simulink model "Modelka_3"  (Simulink 4.00)
settings: Solver=ode45  StartTime=0.0  StopTime=10.0  RelTol=1e-3
settings Model: LastModifiedBy=user

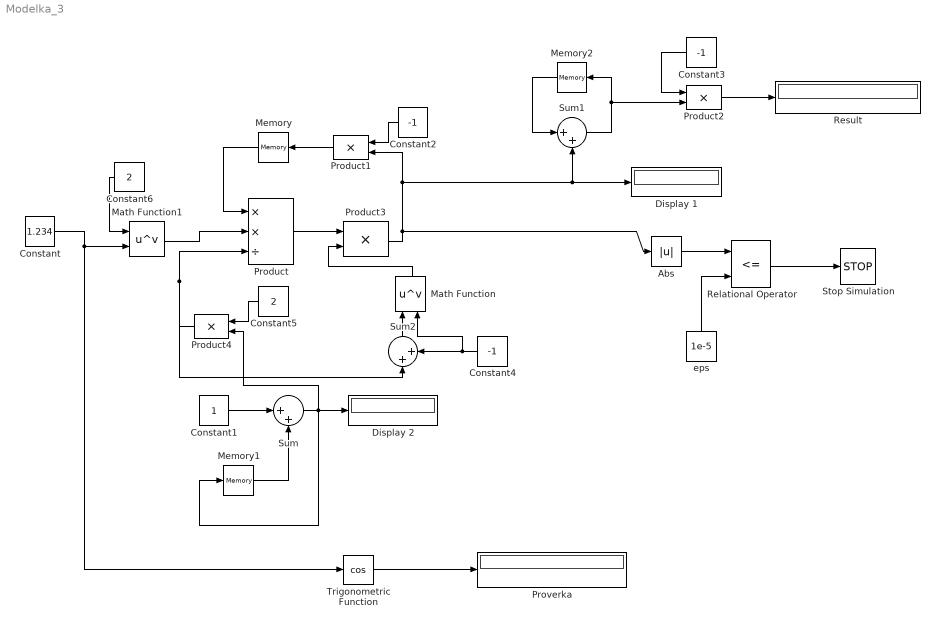
== system Modelka_3 ==
  Abs : Abs  SaturateOnIntegerOverflow=on
  Constant : Constant  Value=1.234
  Constant1 : Constant  Value=1
  Constant2 : Constant  Orientation=left  Value=-1
  Constant3 : Constant  Orientation=left  Value=-1
  Constant4 : Constant  Orientation=left  Value=-1
  Constant5 : Constant  Orientation=left  Value=2
  Constant6 : Constant  Orientation=left  Value=2
  Display 1 : Display
      settings: Format=short
  Display 2 : Display
      settings: Format=short
  Math Function : Math  Orientation=up  Operator=pow  OutputSignalType=auto
  Math Function1 : Math  Operator=pow  OutputSignalType=auto
  Memory : Memory  Orientation=left  X0=1.234  InheritSampleTime=off
      settings: RTWStateStorageClass=Auto
  Memory1 : Memory  X0=0  InheritSampleTime=off
      settings: RTWStateStorageClass=Auto
  Memory2 : Memory  Orientation=left  X0=0  InheritSampleTime=off
      settings: RTWStateStorageClass=Auto
  Product : Product  Inputs=**/  Multiplication=Element-wise(.*)  SaturateOnIntegerOverflow=on
  Product1 : Product  Orientation=left  Inputs=2  Multiplication=Element-wise(.*)  SaturateOnIntegerOverflow=on
  Product2 : Product  Inputs=2  Multiplication=Element-wise(.*)  SaturateOnIntegerOverflow=on
  Product3 : Product  Inputs=2  Multiplication=Element-wise(.*)  SaturateOnIntegerOverflow=on
  Product4 : Product  Orientation=left  Inputs=2  Multiplication=Element-wise(.*)  SaturateOnIntegerOverflow=on
  Proverka : Display
  Relational Operator : RelationalOperator  Operator=<=
  Result : Display
  Stop Simulation : Stop
  Sum : Sum  Inputs=|++  SaturateOnIntegerOverflow=on
  Sum1 : Sum  Inputs=|++  SaturateOnIntegerOverflow=on
  Sum2 : Sum  Orientation=up  Inputs=|++  SaturateOnIntegerOverflow=on
  Trigonometric Function : Trigonometry  Operator=cos  OutputSignalType=auto
  eps : Constant  Orientation=up  Value=1e-5
  wires:
  Memory/1 -> Product/1
  Constant1/1 -> Sum/1
  Memory1/1 -> Sum/2
  Sum/1 -> Display 2/1, Memory1/1, Product4/2
  Sum1/1 -> Memory2/1, Product2/2
  Memory2/1 -> Sum1/1
  Abs/1 -> Relational Operator/1
  eps/1 -> Relational Operator/2
  Relational Operator/1 -> Stop Simulation/1
  Trigonometric Function/1 -> Proverka/1
  Product1/1 -> Memory/1
  Constant2/1 -> Product1/1
  Constant3/1 -> Product2/1
  Product2/1 -> Result/1
  Constant/1 -> Trigonometric Function/1, Math Function1/2
  Constant4/1 -> Sum2/2, Math Function/2
  Product3/1 -> Abs/1, Product1/2, Display 1/1, Sum1/2
  Constant5/1 -> Product4/1
  Product4/1 -> Product/3, Sum2/1
  Sum2/1 -> Math Function/1
  Math Function/1 -> Product3/2
  Product/1 -> Product3/1
  Math Function1/1 -> Product/2
  Constant6/1 -> Math Function1/1
